simulink model "Speed_Control_Model_softStart"  (R2024b)
settings: Solver=VariableStepAuto  StartTime=0  StopTime=1.5*4  FixedStep=1e-6  RelTol=1e-3
libraries: spsDiodeLib x6, spsMosfetLib x5, spsSeriesRLCBranchLib x5, spsPWMGeneratorDCDCLib x4, spsControlledVoltageSourceLib x3, spsVoltageMeasurementLib x3, spsDCMachineLib x2, spsDCVoltageSourceLib x2, spsMeanLib x2, slpidlib x2, simulink x2, spsCurrentMeasurementLib x1
settings Model: SimulationMode=rapid-accelerator  Creator=06MBC93  LastModifiedBy=kamer
settings RTWCC: GPUComputeCapability=3.5

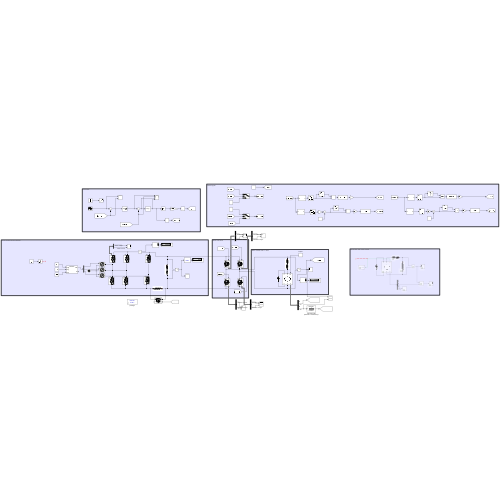
[thumbnail: Simulink's stored preview of the top-level diagram]
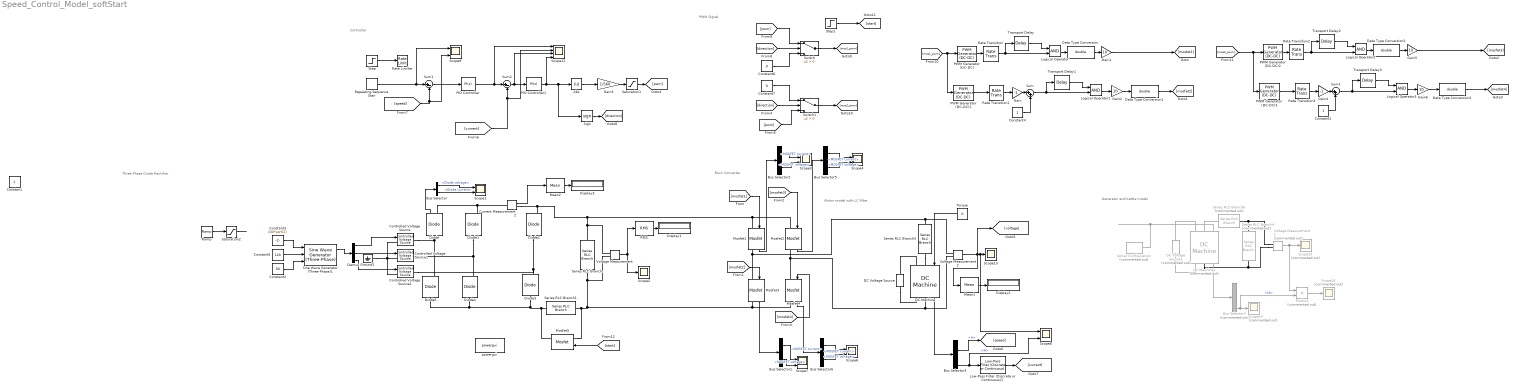
== system Speed_Control_Model_softStart ==
  note: Three Phase Diode Rectifier
  note: Generator and Kettle model
  note: Motor model with LC filter
  note: Buck Converter
  note: PWM Signal
  note: Controller
  Abs : Abs  SaturateOnIntegerOverflow=off
  Bus Selector : BusSelector  OutputSignals=Diode voltage,Diode current
  Bus Selector{1..2,5..6} (4 alike) : BusSelector  OutputSignals=MOSFET current,MOSFET voltage
  Bus Selector3 : BusSelector  OutputSignals=Te,w,iF,iA
  Bus Selector4 : BusSelector  Commented=on  OutputSignals=Te,w,iF,iA
  Constant1 : Constant
  Constant2 : Constant  Value=50
  Constant3 : Constant  Value=230*sqrt(2)
  Constant4 : Constant
  Constant5 : Constant  Value=120
  Constant6 : Constant  Value=0
  Constant7 : Constant  Value=0
  Controlled Voltage Source : spsControlledVoltageSourceLib/Controlled Voltage Source  Initialize=on  Source_Type=DC  Amplitude=0  Phase=0  Frequency=50  Measurements=None
  Controlled Voltage Source1 : spsControlledVoltageSourceLib/Controlled Voltage Source  Initialize=on  Source_Type=DC  Amplitude=0  Phase=120  Frequency=50  Measurements=None
  Controlled Voltage Source2 : spsControlledVoltageSourceLib/Controlled Voltage Source  Initialize=on  Source_Type=DC  Amplitude=0  Phase=240  Frequency=50  Measurements=None
  Current Measurement2 : spsCurrentMeasurementLib/Current Measurement  PhasorSimulation=off  OutputType=Complex  PSBequivalent=0
  DC Machine : spsDCMachineLib/DC Machine  PresetModel=No  MechanicalLoad=Torque TL  FieldType=Wound  ShowDetailedParameters=on  MeasurementBus=on  RLa="[ 0.8  0.0125]"  RLf="[ 210  23]"  Laf=0.482  MachineConstant=Torque constant (N.m/A)  Ke=1.8  Kt=1.8  J=0.12  Bm=0.03  Tf=0.13  w0=0  Ifinit=1.04761904756944  TsPowergui=0  TsBlock=-1
  DC Machine1 : spsDCMachineLib/DC Machine  Commented=on  PresetModel=No  MechanicalLoad=Mechanical rotational port  FieldType=Wound  ShowDetailedParameters=on  MeasurementBus=on  RLa="[ 0.8  0.0125]"  RLf="[ 210  23]"  Laf=0.482  MachineConstant=Torque constant (N.m/A)  Ke=1.8  Kt=1.8  J=0.12  Bm=0.03  Tf=0.13  w0=0  Ifinit=1.04761904761905  TsPowergui=0  TsBlock=-1
  DC Voltage Source : spsDCVoltageSourceLib/DC Voltage Source  Amplitude=220  Measurements=None
  DC Voltage Source1 : spsDCVoltageSourceLib/DC Voltage Source  Commented=on  Amplitude=220  Measurements=None
  Data Type Conversion{,1..3} (4 alike) : DataTypeConversion  OutDataTypeStr=double  SaturateOnIntegerOverflow=off  RndMeth=Floor
  Demux : Demux  Outputs=3
  Diode{,1..5} (6 alike) : spsDiodeLib/Diode  Ron=0.0168  Lon=0  Vf=1  IC=0  UseSnubber=0  Rs=5000  Cs=250e-9  Measurements=on
  Display1 : Display
  Display2 : Display
  Display3 : Display
  Gain : Gain  Gain=-1
  Gain{1..2,5..6} (4 alike) : Gain  Gain=10
  Gain3 : Gain  Gain=1/560
  Gain4 : Gain  Gain=-1
  Ground1 : spsGroundLib/Ground  LConnTagsString=a
  Logical Operator{,1..3} (4 alike) : Logic  AllPortsSameDT=off  OutDataTypeStr=boolean
  Low-Pass Filter (Discrete or Continuous)1 : eeGeneralControl/Low-Pass Filter (Discrete or Continuous)  K=1  T=0.008  B=inf  A=-inf  init_option=Inherited from block input  x0=0  Ts=-1
  Mean1 : spsMeanLib/Mean  Freq=60  Vinit=0  Ts=0
  Mean2 : spsMeanLib/Mean  Freq=60  Vinit=0  Ts=0
  Mosfet{1..5} (5 alike) : spsMosfetLib/Mosfet  Ron=0.001  Lon=0  Rd=0.01  Vfd=0.7  IC=0  Rs=1e5  Cs=inf  Measurements=on
  PID Controller : slpidlib/PID Controller  Controller=PI  Form=Parallel  TimeDomain=Discrete-time  UseExternalTs=off  SampleTime=1/1000  IntegratorMethod=Forward Euler  FilterMethod=Forward Euler  ControllerParametersSource=internal  P=15  I=0.15  UseKiTs=on  D=0.001  UseExternalDerivativeSource=off  N=100  UseFilter=on  TunerSelectOption=Transfer Function Based (PID Tuner App)  InitialConditionSource=internal  InitialConditionForIntegrator=0  InitialConditionForFilter=0  DifferentiatorICPrevScaledInput=0  ExternalReset=none  TrackingMode=off  Kt=1  LimitOutput=on  SatLimitsSource=internal  UpperSaturationLimit=20  LowerSaturationLimit=-20  LinearizeAsGain=on  AntiWindupMode=clamping  Kb=1  LimitIntegrator=off  UpperIntegratorSaturationLimit=inf  LowerIntegratorSaturationLimit=-inf  POutMin=[]  POutMax=[]  IOutMin=[]  IOutMax=[]  DOutMin=[]  DOutMax=[]  NOutMin=[]  NOutMax=[]  SumOutMin=[]  SumOutMax=[]  SaturationOutMin=[]  SaturationOutMax=[]  PParamMin=[]  PParamMax=[]  IParamMin=[]  IParamMax=[]  DParamMin=[]  DParamMax=[]  NParamMin=[]  NParamMax=[]  KbParamMin=[]  KbParamMax=[]  KtParamMin=[]  KtParamMax=[]  KbOutMin=[]  KbOutMax=[]  KtOutMin=[]  KtOutMax=[]  IntegratorOutMin=[]  IntegratorOutMax=[]  FilterOutMin=[]  FilterOutMax=[]  SumI1OutMin=[]  SumI1OutMax=[]  SumI2OutMin=[]  SumI2OutMax=[]  SumI3OutMin=[]  SumI3OutMax=[]  SumI4OutMin=[]  SumI4OutMax=[]  SumDOutMin=[]  SumDOutMax=[]  DifferentiatorOutMin=[]  DifferentiatorOutMax=[]  FilterDiffOutCoefMin=[]  FilterDiffOutCoefMax=[]  ReciprocalOutMin=[]  ReciprocalOutMax=[]  SumDenOutMin=[]  SumDenOutMax=[]  SumNumOutMin=[]  SumNumOutMax=[]  DivideOutMin=[]  DivideOutMax=[]  UdiffTsProdOutMin=[]  UdiffTsProdOutMax=[]  NTsProdOutMin=[]  NTsProdOutMax=[]  UintegralTsProdOutMin=[]  UintegralTsProdOutMax=[]  UngainTsProdOutMin=[]  UngainTsProdOutMax=[]  ClampingZeroOutDataTypeStr=Inherit: Inherit via back propagation  ClampingZeroOutMin=[]  ClampingZeroOutMax=[]  FilterDenConstantOutDataTypeStr=Inherit: Inherit via back propagation  FilterDenConstantOutMin=[]  FilterDenConstantOutMax=[]  PCopyOutDataTypeStr=Inherit: Inherit via back propagation  PCopyOutMin=[]  PCopyOutMax=[]  NCopyOutDataTypeStr=Inherit: Inherit via back propagation  NCopyOutMin=[]  NCopyOutMax=[]  IntegratorContinuousStateAttributes=''  IntegratorStateMustResolveToSignalObject=off  IntegratorRTWStateStorageClass=Auto  FilterContinuousStateAttributes=''  FilterStateMustResolveToSignalObject=off  FilterRTWStateStorageClass=Auto  ParallelPVariant=InternalParameters  IdealPVariant=Disabled  IVariant=InternalParameters  DVariant=Disabled  IntegratorVariant=Discrete  SatVariant=Enabled  AWVariant=DiscClampingParallel  PCopyVariant=Disabled  TRVariant=Disabled  FdbkBlocksVariant=Forward  IdealPFdbkVariant=Disabled  SatFdbkVariant=Disabled  DerivativeFilterVariant=Disabled  NVariant=Disabled  NCopyVariant=Disabled_SignalSpec  FilterICVariant=Disabled  IntegratorICVariant=InternalICs  ExternalResetVariant=Disabled  TRSumVariant=Passthrough  SumFdbkVariant=Disabled  SumVariant=Sum_PI  TsampFilterVariant=InternalTs  TsampNgainVariant=Passthrough  TsampIntegralVariant=Disabled_SignalSpec  ExternalSaturationOutDataTypeStr=Inherit: Same as second input  DerivativeSourceVariant=Disabled  PreIntVariant=InternalPreInt
  PID Controller1 : slpidlib/PID Controller  Controller=PI  Form=Parallel  TimeDomain=Discrete-time  UseExternalTs=off  SampleTime=1/5000  IntegratorMethod=Forward Euler  FilterMethod=Forward Euler  ControllerParametersSource=internal  P=3  I=0.001  UseKiTs=on  D=0  UseExternalDerivativeSource=off  N=100  UseFilter=on  TunerSelectOption=Transfer Function Based (PID Tuner App)  InitialConditionSource=internal  InitialConditionForIntegrator=0  InitialConditionForFilter=0  DifferentiatorICPrevScaledInput=0  ExternalReset=none  TrackingMode=off  Kt=1  LimitOutput=off  SatLimitsSource=internal  UpperSaturationLimit=20  LowerSaturationLimit=-20  LinearizeAsGain=on  AntiWindupMode=clamping  Kb=1  LimitIntegrator=off  UpperIntegratorSaturationLimit=inf  LowerIntegratorSaturationLimit=-inf  POutMin=[]  POutMax=[]  IOutMin=[]  IOutMax=[]  DOutMin=[]  DOutMax=[]  NOutMin=[]  NOutMax=[]  SumOutMin=[]  SumOutMax=[]  SaturationOutMin=[]  SaturationOutMax=[]  PParamMin=[]  PParamMax=[]  IParamMin=[]  IParamMax=[]  DParamMin=[]  DParamMax=[]  NParamMin=[]  NParamMax=[]  KbParamMin=[]  KbParamMax=[]  KtParamMin=[]  KtParamMax=[]  KbOutMin=[]  KbOutMax=[]  KtOutMin=[]  KtOutMax=[]  IntegratorOutMin=[]  IntegratorOutMax=[]  FilterOutMin=[]  FilterOutMax=[]  SumI1OutMin=[]  SumI1OutMax=[]  SumI2OutMin=[]  SumI2OutMax=[]  SumI3OutMin=[]  SumI3OutMax=[]  SumI4OutMin=[]  SumI4OutMax=[]  SumDOutMin=[]  SumDOutMax=[]  DifferentiatorOutMin=[]  DifferentiatorOutMax=[]  FilterDiffOutCoefMin=[]  FilterDiffOutCoefMax=[]  ReciprocalOutMin=[]  ReciprocalOutMax=[]  SumDenOutMin=[]  SumDenOutMax=[]  SumNumOutMin=[]  SumNumOutMax=[]  DivideOutMin=[]  DivideOutMax=[]  UdiffTsProdOutMin=[]  UdiffTsProdOutMax=[]  NTsProdOutMin=[]  NTsProdOutMax=[]  UintegralTsProdOutMin=[]  UintegralTsProdOutMax=[]  UngainTsProdOutMin=[]  UngainTsProdOutMax=[]  ClampingZeroOutDataTypeStr=Inherit: Inherit via back propagation  ClampingZeroOutMin=[]  ClampingZeroOutMax=[]  FilterDenConstantOutDataTypeStr=Inherit: Inherit via back propagation  FilterDenConstantOutMin=[]  FilterDenConstantOutMax=[]  PCopyOutDataTypeStr=Inherit: Inherit via back propagation  PCopyOutMin=[]  PCopyOutMax=[]  NCopyOutDataTypeStr=Inherit: Inherit via back propagation  NCopyOutMin=[]  NCopyOutMax=[]  IntegratorContinuousStateAttributes=''  IntegratorStateMustResolveToSignalObject=off  IntegratorRTWStateStorageClass=Auto  FilterContinuousStateAttributes=''  FilterStateMustResolveToSignalObject=off  FilterRTWStateStorageClass=Auto  ParallelPVariant=InternalParameters  IdealPVariant=Disabled  IVariant=InternalParameters  DVariant=Disabled  IntegratorVariant=Discrete  SatVariant=Disabled  AWVariant=Passthrough  PCopyVariant=Disabled  TRVariant=Disabled  FdbkBlocksVariant=Forward  IdealPFdbkVariant=Disabled  SatFdbkVariant=Disabled  DerivativeFilterVariant=Disabled  NVariant=Disabled  NCopyVariant=Disabled_SignalSpec  FilterICVariant=Disabled  IntegratorICVariant=InternalICs  ExternalResetVariant=Disabled  TRSumVariant=Passthrough  SumFdbkVariant=Disabled  SumVariant=Sum_PI  TsampFilterVariant=InternalTs  TsampNgainVariant=Passthrough  TsampIntegralVariant=Disabled_SignalSpec  ExternalSaturationOutDataTypeStr=Inherit: Same as second input  DerivativeSourceVariant=Disabled  PreIntVariant=InternalPreInt
  PWM Generator (DC-DC){,1..3} (4 alike) : spsPWMGeneratorDCDCLib/PWM Generator (DC-DC)  Fsw=25000  Ts=0
  Product : Product  Commented=on
  RMS : spsRMSLib/RMS  TrueRMS=on  Freq=300  RMSInit=0  Ts=0
  Ramp : simulink/Sources/Ramp  slope=230*sqrt(2)*5  start=0  InitialOutput=0
  Rate Limiter : RateLimiter  RisingSlewLimit=150  FallingSlewLimit=-150  SampleTimeMode=inherited
  Rate Transition{,1..3} (4 alike) : RateTransition  OutPortSampleTime=1e-6
  Repeating Sequence Stair : simulink/Sources/Repeating Sequence Stair  OutValues=[0 30 -30 0].'  tsamp=1.5  OutMin=[]  OutMax=[]  OutDataTypeStr=double  OutputDataTypeScalingMode=double  OutDataType=fixdt(0,8)  ConRadixGroup=Best Precision: Vector-wise  OutScaling=2^-12
  Saturation1 : Saturate  UpperLimit=0.32  LowerLimit=0
  Saturation2 : Saturate  UpperLimit=230*sqrt(2)  LowerLimit=0
  Scope{1,3..4,6..9} (7 alike) : Scope  NumInputPorts=2
  Scope11 : Scope  NumInputPorts=4
  Scope13 : Scope
  Scope14 : Scope  Commented=on
  Scope15 : Scope  Commented=on
  Scope16 : Scope  Commented=on
  Scope2 : Scope
  Series RLC Branch : spsSeriesRLCBranchLib/Series RLC Branch  LConnTagsString=__new0  RConnTagsString=__new0  BranchType=RC  Resistance=5.1e-3  Inductance=3e-3  SetiL0=off  InitialCurrent=0  Capacitance=100e-6  Setx0=off  InitialVoltage=0  Measurements=None
  Series RLC Branch1 : spsSeriesRLCBranchLib/Series RLC Branch  LConnTagsString=__new0  RConnTagsString=__new0  BranchType=R  Resistance=100  Inductance=3e-3  SetiL0=off  InitialCurrent=0  Capacitance=140e-5  Setx0=off  InitialVoltage=0  Measurements=None
  Series RLC Branch3 : spsSeriesRLCBranchLib/Series RLC Branch  LConnTagsString=__new0  RConnTagsString=__new0  BranchType=RL  Resistance=0.27  Inductance=12e-3  SetiL0=off  InitialCurrent=0  Capacitance=70e-6*4  Setx0=off  InitialVoltage=0  Measurements=None
  Series RLC Branch4 : spsSeriesRLCBranchLib/Series RLC Branch  Commented=on  LConnTagsString=__new0  RConnTagsString=__new0  BranchType=R  Resistance=6  Inductance=12e-3  SetiL0=off  InitialCurrent=0  Capacitance=70e-6*4  Setx0=off  InitialVoltage=0  Measurements=None
  Series RLC Branch6 : spsSeriesRLCBranchLib/Series RLC Branch  Commented=on  LConnTagsString=__new0  RConnTagsString=__new0  BranchType=RL  Resistance=0.27  Inductance=12e-3  SetiL0=off  InitialCurrent=0  Capacitance=70e-6*4  Setx0=off  InitialVoltage=0  Measurements=None
  Sign : Signum
  Sine Wave Generator (Three-Phase)1 : eeSinGeneratorThreePhase/Sine Wave Generator (Three-Phase)  Ts=-1
      settings: LibrarySourceBlock=|
      | ee_sl_lib/General Control/Sine Wave Generator
      | (Three-Phase)
  Solver Configuration : nesl_utility/Solver Configuration  Commented=on  PhysicalDomain=network_engine_domain  SubClassName=solver  LeftPortType=input  RightPortType=generic  Tones=[]  Harmonics=[]  SimulateNoise=off  Profile=off  UseLocalSampling=off  EnableSwitchedLinearOptims=on  FrequencyDomain=off  UseCCode=off  RelTol=0.001  AbsTol=0.001  MinStep=1e-09  ToWorkspace=off  RevertToSquareIcSolve=off  NumHomotopyIterations=100  PhasorMode=off  PhasorModeNumHarmonics=1  ConsistencySolver=NEWTON_XTOL_AFTER_FTOL  IndexReductionMethod=DerivativeReplacement  DoDC=off  ResidualTolerance=1e-09  ConsistencyTolSource=GLOBAL  ConsistencyAbsTol=0.001  ConsistencyRelTol=0.001  ConsistencyTolFactor=0.001  UseLocalSolver=off  LocalSolverChoice=NE_BACKWARD_EULER_ADVANCER  ResolveIndetEquations=on  FunctionEvalNumThread=1  LocalSolverSampleTime=0.001  DoFixedCost=off  MaxNonlinIter=3  MaxModeIter=2  ComputeImpulses=off  ImpulseIterations=2  LinearAlgebra=auto  LinearAlgebraNumThread=0  EquationFormulation=NE_TIME_EF  DelaysMemoryBudget=1024  AutomaticFiltering=on  FilteringTimeConstant=0.001  PartitionStorageMethod=AS_NEEDED  PartitionMemoryBudget=1024  PartitionMethod=ROBUST  MultibodyUseLocalSolver=off  MultibodyLocalSolverChoice=ODE1  MultibodyLocalSolverSampleTime=0.001
  Step : Step  Time=0.2  After=20  SampleTime=0
  Step1 : Step  After=20  SampleTime=0
  Sum : Sum  Inputs=|++
  Sum1 : Sum  Inputs=|+-
  Sum2 : Sum  Inputs=|+-
  Sum3 : Sum  Inputs=|++
  Switch : Switch  Criteria=u2 > Threshold  SaturateOnIntegerOverflow=off  InputSameDT=off
  Switch1 : Switch  Criteria=u2 > Threshold  SaturateOnIntegerOverflow=off  InputSameDT=off
  Torque : Constant  Value=0
  Transport Delay{,1..3} (4 alike) : TransportDelay  DelayTime=1/1000000  BufferSize=16384
  Voltage Measurement : spsVoltageMeasurementLib/Voltage Measurement  PhasorSimulation=off  OutputType=Complex  PSBequivalent=0
  Voltage Measurement1 : spsVoltageMeasurementLib/Voltage Measurement  Commented=on  PhasorSimulation=off  OutputType=Complex  PSBequivalent=0
  Voltage Measurement2 : spsVoltageMeasurementLib/Voltage Measurement  PhasorSimulation=off  OutputType=Complex  PSBequivalent=0
  powergui : sps_lib/powergui  Priority=1  SimulationMode=Discrete  SampleTime=1e-6  frequency=60  Iterations=50  frequencyindice=0  Pbase=100e6  ErrMax=1e-4  UnitsV=kV  UnitsW=MW  buscounter=0  FunctionMessages=off  echomessages=off  EnableUseOfTLC=off  CurrentSourceSwitches=off  DisableSnubberDevices=off  DisableRonSwitches=off  DisableVfSwitches=off  DisplayEquations=off  AutomaticDiscreteSolvers=off  SolverType=Tustin/Backward Euler (TBE)  Interpol=off  ExternalGateDelay=off  methode=off  Ts=100  x0status=blocks  SPID=on  SwTol=0  HookPort=off  NonlinearTolerance=1e-4  nMaxIteration=100  ContinueOnMaxIteration=off  RestoreLinks=warning  ResistiveCurrentMeasurement=off  Frange=[0:2:500]  Ylog=off  Xlog=on  ShowGrid=off  save=off  variable=ZData  structure=0  ZoomFFT=off  StartTime=0.0  cycles=1  DisplayStyle=1  fundamental=60  FreqAxis=off  MaxFrequency=1000  frequencyindicesteady=1  RmsSteady=1  display=off
  Constan1 : Constant  IOType=siggen
  wires:
  Voltage Measurement/1 -> Scope2/1, RMS/1
  RMS/1 -> Display1/1
  Diode/1 -> Bus Selector/1
  Bus Selector/2 -> Scope1/2  "<Diode current>"
  Bus Selector/1 -> Scope1/1  "<Diode voltage>"
  Voltage Measurement2/1 -> Scope8/1, Scope13/1, [voltage], Mean1/1
  Mean1/1 -> Display2/1
  Current Measurement2/1 -> Mean2/1
  Mean2/1 -> Display3/1
  [mosfet2] -> Mosfet3/1
  DC Machine/1 -> Bus Selector3/1
  Bus Selector3/4 -> Low-Pass Filter (Discrete or Continuous)1/1, Scope8/2  "<iA>"
  Constant4/1 -> Sum/2
  Gain/1 -> Sum/1
  Transport Delay/1 -> Logical Operator/1
  PWM Generator (DC-DC)/1 -> Rate Transition/1
  Sum/1 -> Logical Operator1/2, Transport Delay1/1
  Transport Delay1/1 -> Logical Operator1/1
  Logical Operator1/1 -> Gain2/1
  Logical Operator/1 -> Data Type Conversion/1
  Data Type Conversion/1 -> Gain1/1
  Data Type Conversion1/1 -> [mosfet2]
  [mosfet1] -> Mosfet1/1
  [mosfet3] -> Mosfet2/1
  [mosfet4] -> Mosfet4/1
  Gain2/1 -> Data Type Conversion1/1
  Gain1/1 -> [mosfet1]
  Rate Transition/1 -> Logical Operator/2, Transport Delay/1
  Rate Transition1/1 -> Gain/1
  [speed] -> Scope9/2, Sum1/2
  PID Controller/1 -> Scope11/1, Sum2/1
  [current] -> Scope11/2, Sum2/2
  Sum2/1 -> Scope11/3, PID Controller1/1
  Sum1/1 -> PID Controller/1
  Step/1 -> Rate Limiter/1
  DC Machine1/1 -> Bus Selector4/1
  Bus Selector4/4 -> Product/2, Scope14/1  "<iA>"
  Voltage Measurement1/1 -> Product/1, Scope15/1
  Product/1 -> Scope16/1
  Gain5/1 -> [mosfet3]
  PWM Generator (DC-DC)1/1 -> Rate Transition1/1
  Bus Selector3/2 -> [speed]  "<w>"
  Torque/1 -> DC Machine/1
  PID Controller1/1 -> Scope11/4, Sign/1, Abs/1
  Gain3/1 -> Saturation1/1
  Repeating Sequence Stair/1 -> Scope9/1, Sum1/1
  Saturation1/1 -> [pwm]
  [mos1_pwm] -> PWM Generator (DC-DC)1/1, PWM Generator (DC-DC)/1
  Ramp/1 -> Saturation2/1
  Constant5/1 -> Sine Wave Generator (Three-Phase)1/2
  Constant2/1 -> Sine Wave Generator (Three-Phase)1/3
  Sine Wave Generator (Three-Phase)1/1 -> Demux/1
  Demux/2 -> Controlled Voltage Source1/1
  Demux/3 -> Controlled Voltage Source2/1
  Demux/1 -> Controlled Voltage Source/1
  Saturation2/1 -> ?
  Mosfet3/1 -> Bus Selector1/1
  Mosfet2/1 -> Bus Selector5/1
  Mosfet1/1 -> Bus Selector2/1
  Mosfet4/1 -> Bus Selector6/1
  Bus Selector2/1 -> Scope3/1  "<MOSFET current>"
  Bus Selector2/2 -> Scope3/2  "<MOSFET voltage>"
  Bus Selector5/1 -> Scope4/1  "<MOSFET current>"
  Bus Selector5/2 -> Scope4/2  "<MOSFET voltage>"
  Bus Selector6/1 -> Scope6/1  "<MOSFET current>"
  Bus Selector6/2 -> Scope6/2  "<MOSFET voltage>"
  Bus Selector1/1 -> Scope7/1  "<MOSFET current>"
  Bus Selector1/2 -> Scope7/2  "<MOSFET voltage>"
  Low-Pass Filter (Discrete or Continuous)1/1 -> [current]
  Sign/1 -> [direction]
  [direction] -> Switch/2
  [pwm] -> Switch/1
  Constant6/1 -> Switch/3
  Switch/1 -> [mos1_pwm]
  Switch1/1 -> [mos2_pwm]
  Constant7/1 -> Switch1/1
  [pwm] -> Switch1/3
  [direction] -> Switch1/2
  [mos2_pwm] -> PWM Generator (DC-DC)2/1, PWM Generator (DC-DC)3/1
  PWM Generator (DC-DC)3/1 -> Rate Transition3/1
  Rate Transition3/1 -> Gain4/1
  Rate Transition2/1 -> Transport Delay2/1, Logical Operator2/2
  Gain6/1 -> Data Type Conversion3/1
  Data Type Conversion3/1 -> [mosfet4]
  Data Type Conversion2/1 -> Gain5/1
  Logical Operator2/1 -> Data Type Conversion2/1
  Logical Operator3/1 -> Gain6/1
  Transport Delay3/1 -> Logical Operator3/1
  Sum3/1 -> Transport Delay3/1, Logical Operator3/2
  PWM Generator (DC-DC)2/1 -> Rate Transition2/1
  Transport Delay2/1 -> Logical Operator2/1
  Gain4/1 -> Sum3/1
  Constant1/1 -> Sum3/2
  Abs/1 -> Gain3/1
  Constant3/1 -> Sine Wave Generator (Three-Phase)1/1
  [start] -> Mosfet5/1
  Step1/1 -> [start]
  connections:
  Diode2/LConn1 -- Controlled Voltage Source2/RConn1 -- Diode3/RConn1
  Mosfet1/RConn1 -- Voltage Measurement2/LConn1 -- Series RLC Branch3/LConn1 -- Mosfet3/LConn1
  Diode/RConn1 -- Diode1/RConn1 -- Current Measurement2/LConn1
  Mosfet4/LConn1 -- DC Machine/RConn1 -- Voltage Measurement2/LConn2 -- Mosfet2/RConn1
  DC Voltage Source/LConn1 -- DC Machine/RConn2
  DC Machine/LConn2 -- DC Voltage Source/RConn1
  Series RLC Branch3/RConn1 -- DC Machine/LConn1
  Solver Configuration/RConn1 -- DC Machine1/LConn1
  DC Machine1/LConn3 -- DC Voltage Source1/RConn1
  DC Machine1/RConn2 -- DC Voltage Source1/LConn1
  Voltage Measurement1/LConn1 -- Series RLC Branch6/LConn1 -- Series RLC Branch4/LConn1
  Voltage Measurement1/LConn2 -- DC Machine1/RConn1 -- Series RLC Branch4/RConn1
  Diode2/RConn1 -- Current Measurement2/RConn1 -- Mosfet2/LConn1 -- Mosfet1/LConn1 -- Voltage Measurement/LConn1 -- Series RLC Branch/LConn1
  Diode3/LConn1 -- Mosfet5/RConn1 -- Series RLC Branch1/RConn1 -- Diode4/LConn1 -- Diode5/LConn1
  DC Machine1/LConn2 -- Series RLC Branch6/RConn1
  Diode5/RConn1 -- Controlled Voltage Source/RConn1 -- Diode/LConn1
  Diode1/LConn1 -- Controlled Voltage Source1/RConn1 -- Diode4/RConn1
  Ground1/LConn1 -- Controlled Voltage Source2/LConn1 -- Controlled Voltage Source1/LConn1 -- Controlled Voltage Source/LConn1
  Mosfet3/RConn1 -- Mosfet4/RConn1 -- Series RLC Branch/RConn1 -- Voltage Measurement/LConn2 -- Mosfet5/LConn1 -- Series RLC Branch1/LConn1
